simulink model "counter1"  (R2019a)
settings: Solver=FixedStepDiscrete  StartTime=0.0  StopTime=50  FixedStep=1  RelTol=1e-3
settings Model: Creator=vmadmin  LastModifiedBy=vmadmin

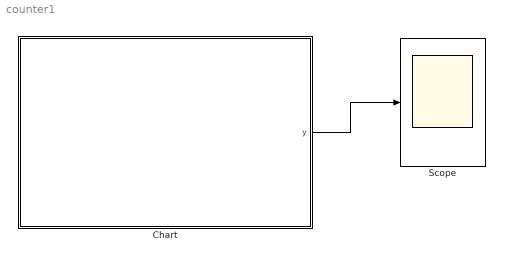
== system counter1 ==
  Chart : Stateflow chart  BlockKeywords=__PRM__SERIALIZED__DATA__:Stateflow Chart,Stateflow Diagram  TreatAsAtomicUnit=on
  Scope : Scope
  wires:
  Chart/1(y) -> Scope/1

== stateflow chart counter1/Chart ==
  state A1
    en:y=0;
    du:y=y+1;
  (default) -> A1 : {y=double(0);}
  A1 -> A1 : [y>=5]
  data: y output double
